simulink model "PicturePicture"  (R2015b)
settings: Solver=VariableStepAuto  StartTime=0.0  StopTime=500  RelTol=1e-3
libraries: simulink x4, powerlib_meascontrol x2
settings Model: Creator=ramin  LastModifiedBy=ramin

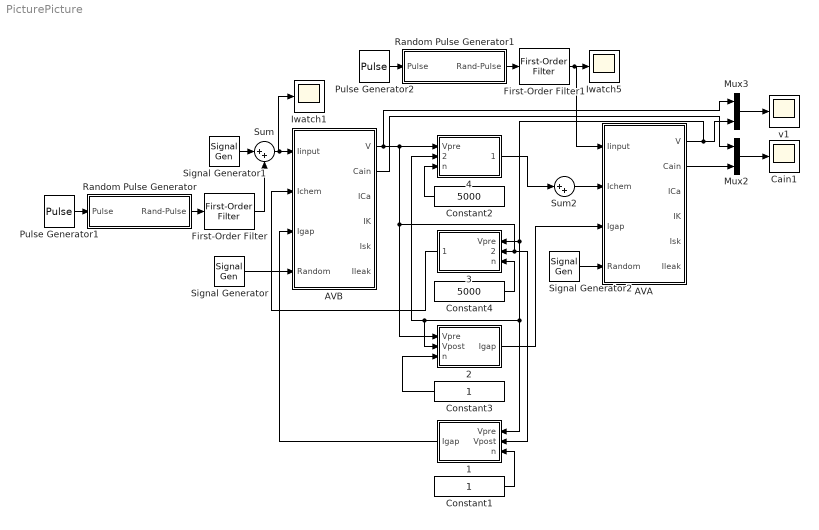
== system PicturePicture ==
  1 : Subsystem
  2 : Subsystem
  3 : Subsystem
  4 : Subsystem
  AVA : Subsystem
  AVB : Subsystem
  Cain1 : Scope
  Constant1 : Constant
  Constant2 : Constant  Value=5000
  Constant3 : Constant
  Constant4 : Constant  Value=5000
  First-Order Filter : powerlib_meascontrol/Filters/First-Order Filter  FilterType=Lowpass  Tc=1  Ts=0  Initialize=off  Vac_Init=[0, 0, 60]  Vdc_Init=0  PlotResponse=off  FreqRange="[0,  200,  1]"
  First-Order Filter1 : powerlib_meascontrol/Filters/First-Order Filter  FilterType=Lowpass  Tc=1  Ts=0  Initialize=off  Vac_Init=[0, 0, 60]  Vdc_Init=0  PlotResponse=off  FreqRange="[0,  200,  1]"
  Iwatch1 : Scope
  Iwatch5 : Scope
  Mux2 : Mux  Inputs=2
  Mux3 : Mux  Inputs=2
  Pulse Generator1 : DiscretePulseGenerator  PulseType=Time based  Amplitude=2000  Period=200  PulseWidth=80  PhaseDelay=2
  Pulse Generator2 : DiscretePulseGenerator  PulseType=Time based  Amplitude=2000  Period=200  PulseWidth=80  PhaseDelay=2
  Random Pulse Generator : Subsystem
  Random Pulse Generator1 : Subsystem
  Signal Generator : SignalGenerator  WaveForm=random  Amplitude=0.5  Frequency=100
  Signal Generator1 : SignalGenerator  WaveForm=random  Amplitude=0  Frequency=100
  Signal Generator2 : SignalGenerator  WaveForm=random  Amplitude=0.5  Frequency=100
  Sum : Sum  Inputs=|++
  Sum2 : Sum  Inputs=|++
  v1 : Scope
  wires:
  Signal Generator/1 -> AVB/4(Random)
  Signal Generator1/1 -> Sum/1
  Signal Generator2/1 -> AVA/4(Random)
  Constant2/1 -> 4/3(n)
  Constant3/1 -> 2/3(n)
  AVA/1(V) -> 1/1(Vpre), 2/2(Vpost), 4/2(Vpost), 3/1(Vpre), Mux3/2
  Sum/1 -> Iwatch1/1, AVB/1(Iinput)
  Random Pulse Generator/1(Rand-Pulse) -> First-Order Filter/1
  Sum2/1 -> AVA/2(Ichem)
  Constant1/1 -> 1/3(n)
  1/1(Igap) -> AVB/3(Igap)
  First-Order Filter1/1 -> AVA/1(Iinput), Iwatch5/1
  3/1(Ichem) -> AVB/2(Ichem)
  2/1(Igap) -> AVA/3(Igap)
  Mux2/1 -> Cain1/1
  Mux3/1 -> v1/1
  AVB/2("Cain ") -> Mux2/1
  4/1(Ichem) -> Sum2/1
  Pulse Generator1/1 -> Random Pulse Generator/1(Pulse)
  AVA/2("Cain ") -> Mux2/2
  Random Pulse Generator1/1(Rand-Pulse) -> First-Order Filter1/1
  Pulse Generator2/1 -> Random Pulse Generator1/1(Pulse)
  Constant4/1 -> 3/3(n)
  AVB/1(V) -> 4/1(Vpre), 2/1(Vpre), 1/2(Vpost), 3/2(Vpost), Mux3/1
  First-Order Filter/1 -> Sum/2

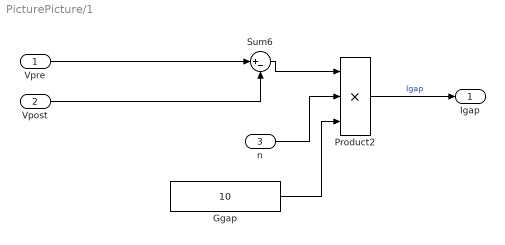
== system PicturePicture/1 ==
  Vpre : Inport
  Vpost : Inport  Port=2
  n : Inport  Port=3
  Ggap : Constant  Value=10
  Product2 : Product  Inputs=3
  Sum6 : Sum  Inputs=|+-
  Igap : Outport
  wires:
  Vpre/1 -> Sum6/1
  n/1 -> Product2/2
  Sum6/1 -> Product2/1
  Product2/1 -> Igap/1  "Igap"
  Vpost/1 -> Sum6/2
  Ggap/1 -> Product2/3

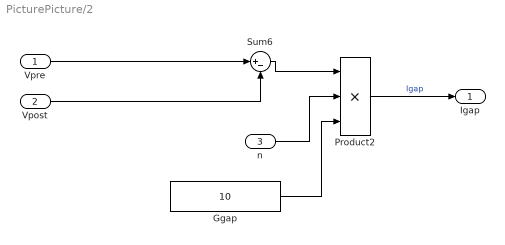
== system PicturePicture/2 ==
  Vpre : Inport
  Vpost : Inport  Port=2
  n : Inport  Port=3
  Ggap : Constant  Value=10
  Product2 : Product  Inputs=3
  Sum6 : Sum  Inputs=|+-
  Igap : Outport
  wires:
  Vpre/1 -> Sum6/1
  n/1 -> Product2/2
  Sum6/1 -> Product2/1
  Product2/1 -> Igap/1  "Igap"
  Vpost/1 -> Sum6/2
  Ggap/1 -> Product2/3

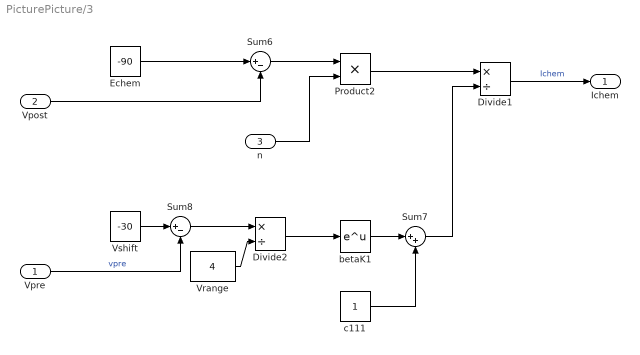
== system PicturePicture/3 ==
  Vpre : Inport
  Vpost : Inport  Port=2
  n : Inport  Port=3
  Divide1 : Product  Inputs=*/
  Divide2 : Product  Inputs=*/
  Echem : Constant  Value=-90
  Product2 : Product
  Sum6 : Sum  Inputs=|+-
  Sum7 : Sum  Inputs=|++
  Sum8 : Sum  Inputs=|+-
  Vrange : Constant  Value=4
  Vshift : Constant  Value=-30
  betaK1 : Math  SaturateOnIntegerOverflow=on
  c111 : Constant
  Ichem : Outport
  wires:
  Echem/1 -> Sum6/1
  n/1 -> Product2/2
  Sum6/1 -> Product2/1
  Product2/1 -> Divide1/1
  betaK1/1 -> Sum7/1
  c111/1 -> Sum7/2
  Vshift/1 -> Sum8/1
  Vpre/1 -> Sum8/2  "vpre"
  Sum8/1 -> Divide2/1
  Vrange/1 -> Divide2/2
  Divide2/1 -> betaK1/1
  Sum7/1 -> Divide1/2
  Divide1/1 -> Ichem/1  "Ichem"
  Vpost/1 -> Sum6/2

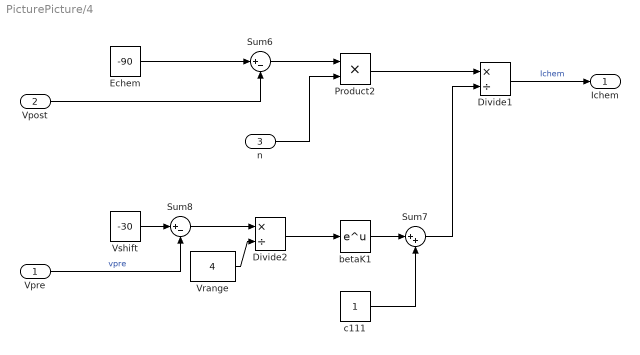
== system PicturePicture/4 ==
  Vpre : Inport
  Vpost : Inport  Port=2
  n : Inport  Port=3
  Divide1 : Product  Inputs=*/
  Divide2 : Product  Inputs=*/
  Echem : Constant  Value=-90
  Product2 : Product
  Sum6 : Sum  Inputs=|+-
  Sum7 : Sum  Inputs=|++
  Sum8 : Sum  Inputs=|+-
  Vrange : Constant  Value=4
  Vshift : Constant  Value=-30
  betaK1 : Math  SaturateOnIntegerOverflow=on
  c111 : Constant
  Ichem : Outport
  wires:
  Echem/1 -> Sum6/1
  n/1 -> Product2/2
  Sum6/1 -> Product2/1
  Product2/1 -> Divide1/1
  betaK1/1 -> Sum7/1
  c111/1 -> Sum7/2
  Vshift/1 -> Sum8/1
  Vpre/1 -> Sum8/2  "vpre"
  Sum8/1 -> Divide2/1
  Vrange/1 -> Divide2/2
  Divide2/1 -> betaK1/1
  Sum7/1 -> Divide1/2
  Divide1/1 -> Ichem/1  "Ichem"
  Vpost/1 -> Sum6/2

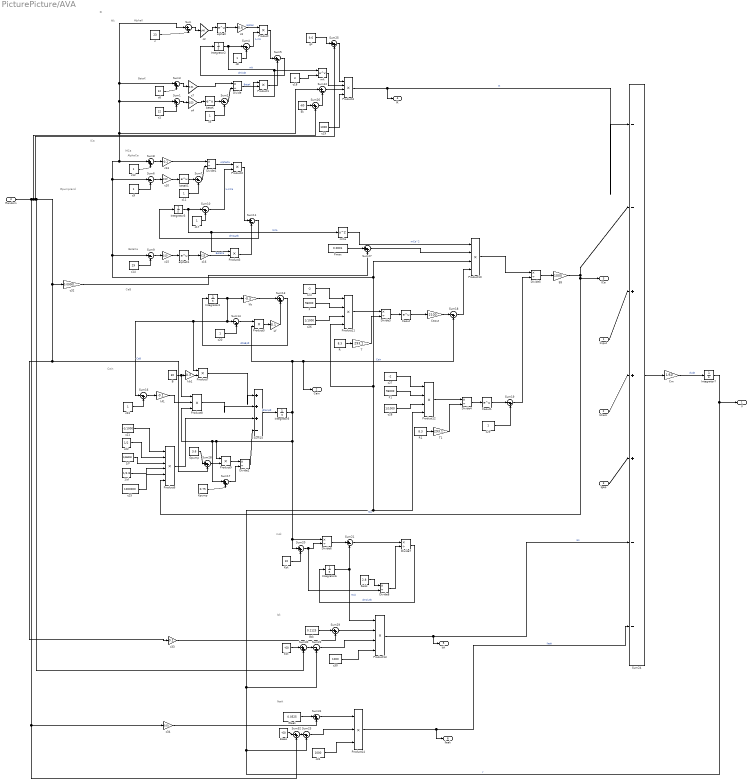
== system PicturePicture/AVA ==
  note: Gpumprand
  note: Isk
  note: msk
  note: ICa
  note: Cain
  note: CaB
  note: BetaCa
  note: AlphaCa
  note: MCa
  note: IK
  note: Mk
  note: BetaK
  note: AlphaK
  note: Ileak
  Iinput : Inport
  Ichem : Inport  Port=2
  Igap : Inport  Port=3
  Random : Inport  Port=4
  1/F : Constant  Value=1/96000
  1/d : Constant  Value=1/2.8
  B : Constant  Value=30
  Caout : Math  SaturateOnIntegerOverflow=on
  "Caout " : Gain  Gain=2100
  Caout1 : Math  SaturateOnIntegerOverflow=on
  "Cm " : Gain  Gain=1/50
  Divide{,1..8} (9 alike) : Product  Inputs=*/
  "Ek " : Constant  Value=-60
  Eleak : Constant  Value=-60
  Esk : Constant  Value=-60
  F : Constant  Value=96000
  F1 : Constant  Value=96000
  Gleak : Constant  Value=0.0525
  Gpump : Constant  Value=3.6
  Gsk : Constant  Value=0.2125
  Integrator2 : Integrator
  Integrator3 : Integrator  InitialCondition=0.001
  Integrator4 : Integrator
  Integrator5 : Integrator
  Integrator6 : Integrator  InitialCondition=1
  Integrator7 : Integrator  InitialCondition=-60
  Kpump : Constant  Value=0.75
  Ksk : Constant  Value=10
  Pmax : Constant  Value=0.0001
  Product{,1..3,5,7,9} (7 alike) : Product
  Product{4,10..13} (5 alike) : Product  Inputs=4
  Product14 : Product  Inputs=3
  Product6 : Product  Inputs=6
  Product8 : Product  Inputs=3
  R : Constant  Value=8.3
  R1 : Constant  Value=8.3
  Saisk : Constant  Value=2.8
  Sum{,2,5,7,11..12,21} (7 alike) : Sum  Inputs=|+-
  Sum{1,3,8,13,17,20,25..32} (14 alike) : Sum  Inputs=|++
  Sum{4,10,14,16,18..19,22..23} (8 alike) : Sum  Inputs=|-+
  Sum15 : Sum  Inputs=|+++-
  Sum24 : Sum  Inputs=|--+++--
  Sum6 : Sum  Inputs=|--
  Sum9 : Sum  Inputs=|--
  T : Gain  Gain=293.1
  T1 : Gain  Gain=293.1
  alphaK : Math  SaturateOnIntegerOverflow=on
  alphaK1 : Math  SaturateOnIntegerOverflow=on
  betaK : Math  SaturateOnIntegerOverflow=on
  betaK1 : Math  SaturateOnIntegerOverflow=on
  c : Constant  Value=23
  c1 : Constant  Value=12
  c10 : Gain  Gain=1/10
  c{5,8..9,11..12,17,20,23,29} (9 alike) : Constant
  c13 : Gain  Gain=-0.2
  c14 : Constant  Value=29
  c15 : Gain  Gain=1/10
  c16 : Gain  Gain=0.23
  c18 : Constant  Value=3
  c19 : Constant  Value=1000
  c2 : Gain  Gain=1/46
  c21 : Constant  Value=-1/1000
  c22 : Constant  Value=1/2
  c24 : Constant  Value=-2
  c25 : Constant  Value=1000000
  c26 : Constant  Value=1/1000
  c27 : Constant  Value=-2
  c28 : Constant  Value=1/1000
  c3 : Gain  Gain=0.6
  c30 : Constant  Value=1000
  c31 : Constant  Value=1000
  c32 : Gain  Gain=0.00001
  c33 : Gain  Gain=0.1
  c34 : Gain  Gain=0.01
  c4 : Gain  Gain=1/23
  c6 : Constant  Value=12
  c7 : Gain  Gain=0.01
  "gg " : Gain  Gain=1000
  gk : Constant  Value=9.6
  kb : Gain  Gain=-0.3
  kb1 : Gain  Gain=0.3
  kf : Gain  Gain=0.1
  kf1 : Gain  Gain=-0.1
  mCa : Math  Operator=square  SaturateOnIntegerOverflow=on
  mk : Math  Operator=pow  SaturateOnIntegerOverflow=on
  V : Outport
  "Cain " : Outport  Port=2
  ICa : Outport  Port=3
  IK : Outport  Port=4
  Isk : Outport  Port=5
  Ileak : Outport  Port=6
  wires:
  Divide/1 -> Product1/2  "BetaK"
  c10/1 -> betaK1/1
  Sum7/1 -> Divide1/2
  c/1 -> Sum/2
  R/1 -> T/1
  c3/1 -> Product/1  "alphaK"
  c9/1 -> Sum6/2
  c6/1 -> Sum3/2
  Product/1 -> Sum5/1
  Sum1/1 -> c4/1
  c13/1 -> Divide1/1
  Caout1/1 -> Sum19/1
  T/1 -> Divide3/2
  Ksk/1 -> Sum20/2
  Product14/1 -> Ileak/1, Sum24/7  "Ileak"
  Sum24/1 -> "Cm "/1
  "Cm "/1 -> Integrator7/1  "dv/dt"
  Divide3/1 -> Caout/1
  c31/1 -> Product14/3
  Integrator6/1 -> Sum21/2, Product13/1  "msk"
  Sum21/1 -> Divide7/1
  Sum23/1 -> Product14/2
  Divide6/1 -> Sum21/1
  c12/1 -> Sum8/2
  Integrator3/1 -> Product3/1, mCa/1, Sum10/1  "mCa"
  Sum5/1 -> Integrator2/1  "dmk/dt"
  c15/1 -> alphaK1/1
  Sum9/1 -> c15/1
  c2/1 -> alphaK/1
  Sum22/1 -> Product13/3
  Product10/1 -> Divide5/1
  Integrator2/1 -> mk/1, Product1/1, Sum4/1  "mk"
  Divide8/1 -> Divide7/2
  R1/1 -> T1/1
  Caout/1 -> "Caout "/1
  Sum3/1 -> c7/1
  Sum6/1 -> c10/1
  Divide4/1 -> Caout1/1
  c30/1 -> Product13/4
  c28/1 -> Product12/3
  c11/1 -> Sum7/2
  betaK1/1 -> Sum7/1
  Divide7/1 -> Integrator6/1  "dmsk/dt"
  Ichem/1 -> Sum24/4
  c7/1 -> Divide/1
  Sum14/1 -> Product5/1
  Sum13/1 -> Integrator4/1  "dCaB/dt"
  Integrator5/1 -> Sum20/1, Divide6/1, Product9/1, Sum17/1, Product8/3, "Cain "/1, Sum18/2, Product5/2  "Cain"
  c21/1 -> Product6/1
  c22/1 -> Product6/2
  1/F/1 -> Product6/3
  1/d/1 -> Product6/4
  c25/1 -> Product6/5
  "gg "/1 -> Sum24/2, ICa/1, Product6/6  "ICa"
  B/1 -> Product8/1, kb1/1
  kb1/1 -> Product7/2
  Product7/1 -> Sum15/1
  Product5/1 -> kf/1
  kf/1 -> Sum13/2
  c23/1 -> Sum16/2
  Sum16/1 -> kf1/1
  kf1/1 -> Product8/2
  Product8/1 -> Sum15/2
  Product6/1 -> Sum15/3
  Product9/1 -> Divide2/1
  Kpump/1 -> Sum17/2
  Sum17/1 -> Divide2/2
  Divide2/1 -> Sum15/4
  Sum15/1 -> Integrator5/1  "dCain/dt"
  mCa/1 -> Product10/1  "mCa^2"
  c24/1 -> Product11/1
  F/1 -> Product11/2
  c26/1 -> Product11/3
  Integrator7/1 -> V/1, Sum22/2, Product11/4, Product10/3, Sum6/1, Sum1/1, Sum3/1, Sum/1, Sum12/1, Sum8/1, Sum9/1, Product12/4, Sum23/2  "v"
  c14/1 -> Sum9/2
  Saisk/1 -> Divide8/1
  Sum18/1 -> Product10/4
  Iinput/1 -> Sum24/3
  "Caout "/1 -> Sum18/1
  Sum/1 -> c2/1
  Sum8/1 -> c13/1
  c16/1 -> Product3/2  "BetaCa"
  Product11/1 -> Divide3/1
  T1/1 -> Divide4/2
  betaK/1 -> Sum2/1
  c29/1 -> Sum19/2
  Product1/1 -> Sum5/2
  c4/1 -> betaK/1
  alphaK/1 -> c3/1
  alphaK1/1 -> c16/1
  Divide1/1 -> Product2/1  "AlphaCa"
  Sum2/1 -> Divide/2
  Sum4/1 -> Product/2  "1-mk"
  c5/1 -> Sum2/2
  c8/1 -> Sum4/2
  Igap/1 -> Sum24/5
  Product13/1 -> Isk/1, Sum24/6  "Isk"
  Divide5/1 -> "gg "/1
  Sum20/1 -> Divide8/2, Divide6/2
  Product12/1 -> Divide4/1
  c27/1 -> Product12/1
  F1/1 -> Product12/2
  c1/1 -> Sum1/2
  Sum11/1 -> Integrator3/1  "dmCa/dt"
  c17/1 -> Sum10/2
  "Ek "/1 -> Sum26/1
  Sum10/1 -> Product2/2  "1-mCa"
  Sum12/1 -> Product4/3
  Product3/1 -> Sum11/2
  Product4/1 -> IK/1, Sum24/1  "IK"
  Integrator4/1 -> Product7/1, Sum16/1, Sum14/1, kb/1  "CaB"
  kb/1 -> Sum13/1
  c20/1 -> Sum14/2
  mk/1 -> Product4/2
  Random/1 -> c32/1, c33/1, Sum28/2, Sum30/2, Sum25/2, Sum26/2, Sum32/2, c34/1
  c19/1 -> Product4/4
  Product2/1 -> Sum11/1
  c18/1 -> mk/2
  Sum19/1 -> Divide5/2
  gk/1 -> Sum25/1
  Sum25/1 -> Product4/1
  Sum26/1 -> Sum12/2
  Pmax/1 -> Sum27/1
  Sum27/1 -> Product10/2
  Sum28/1 -> Product9/2
  Gpump/1 -> Sum28/1
  Sum29/1 -> Product13/2
  Gsk/1 -> Sum29/1
  Sum30/1 -> Sum22/1
  Esk/1 -> Sum30/1
  Gleak/1 -> Sum31/1
  Sum31/1 -> Product14/1
  Sum32/1 -> Sum23/1
  Eleak/1 -> Sum32/1
  c32/1 -> Sum27/2
  c33/1 -> Sum29/2
  c34/1 -> Sum31/2

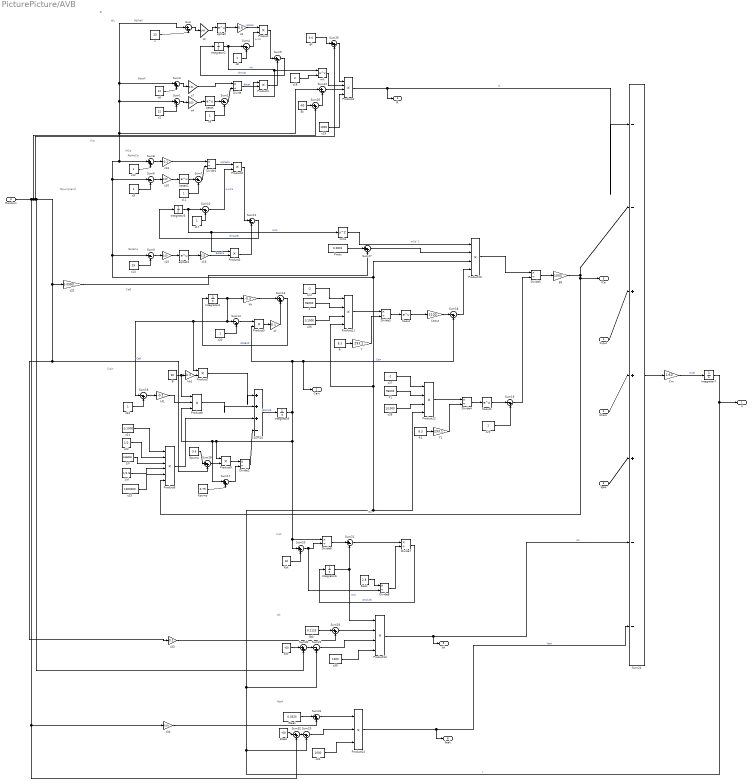
== system PicturePicture/AVB ==
  note: Gpumprand
  note: Isk
  note: msk
  note: ICa
  note: Cain
  note: CaB
  note: BetaCa
  note: AlphaCa
  note: MCa
  note: IK
  note: Mk
  note: BetaK
  note: AlphaK
  note: Ileak
  Iinput : Inport
  Ichem : Inport  Port=2
  Igap : Inport  Port=3
  Random : Inport  Port=4
  1/F : Constant  Value=1/96000
  1/d : Constant  Value=1/2.8
  B : Constant  Value=30
  Caout : Math  SaturateOnIntegerOverflow=on
  "Caout " : Gain  Gain=2100
  Caout1 : Math  SaturateOnIntegerOverflow=on
  "Cm " : Gain  Gain=1/50
  Divide{,1..8} (9 alike) : Product  Inputs=*/
  "Ek " : Constant  Value=-60
  Eleak : Constant  Value=-60
  Esk : Constant  Value=-60
  F : Constant  Value=96000
  F1 : Constant  Value=96000
  Gleak : Constant  Value=0.0525
  Gpump : Constant  Value=3.6
  Gsk : Constant  Value=0.2125
  Integrator2 : Integrator
  Integrator3 : Integrator  InitialCondition=0.001
  Integrator4 : Integrator
  Integrator5 : Integrator
  Integrator6 : Integrator  InitialCondition=1
  Integrator7 : Integrator  InitialCondition=-60
  Kpump : Constant  Value=0.75
  Ksk : Constant  Value=10
  Pmax : Constant  Value=0.0001
  Product{,1..3,5,7,9} (7 alike) : Product
  Product{4,10..13} (5 alike) : Product  Inputs=4
  Product14 : Product  Inputs=3
  Product6 : Product  Inputs=6
  Product8 : Product  Inputs=3
  R : Constant  Value=8.3
  R1 : Constant  Value=8.3
  Saisk : Constant  Value=2.8
  Sum{,2,5,7,11..12,21} (7 alike) : Sum  Inputs=|+-
  Sum{1,3,8,13,17,20,25..32} (14 alike) : Sum  Inputs=|++
  Sum{4,10,14,16,18..19,22..23} (8 alike) : Sum  Inputs=|-+
  Sum15 : Sum  Inputs=|+++-
  Sum24 : Sum  Inputs=|--+++--
  Sum6 : Sum  Inputs=|--
  Sum9 : Sum  Inputs=|--
  T : Gain  Gain=293.1
  T1 : Gain  Gain=293.1
  alphaK : Math  SaturateOnIntegerOverflow=on
  alphaK1 : Math  SaturateOnIntegerOverflow=on
  betaK : Math  SaturateOnIntegerOverflow=on
  betaK1 : Math  SaturateOnIntegerOverflow=on
  c : Constant  Value=23
  c1 : Constant  Value=12
  c10 : Gain  Gain=1/10
  c{5,8..9,11..12,17,20,23,29} (9 alike) : Constant
  c13 : Gain  Gain=-0.2
  c14 : Constant  Value=29
  c15 : Gain  Gain=1/10
  c16 : Gain  Gain=0.23
  c18 : Constant  Value=3
  c19 : Constant  Value=1000
  c2 : Gain  Gain=1/46
  c21 : Constant  Value=-1/1000
  c22 : Constant  Value=1/2
  c24 : Constant  Value=-2
  c25 : Constant  Value=1000000
  c26 : Constant  Value=1/1000
  c27 : Constant  Value=-2
  c28 : Constant  Value=1/1000
  c3 : Gain  Gain=0.6
  c30 : Constant  Value=1000
  c31 : Constant  Value=1000
  c32 : Gain  Gain=0.00001
  c33 : Gain  Gain=0.1
  c34 : Gain  Gain=0.01
  c4 : Gain  Gain=1/23
  c6 : Constant  Value=12
  c7 : Gain  Gain=0.01
  "gg " : Gain  Gain=1000
  gk : Constant  Value=9.6
  kb : Gain  Gain=-0.3
  kb1 : Gain  Gain=0.3
  kf : Gain  Gain=0.1
  kf1 : Gain  Gain=-0.1
  mCa : Math  Operator=square  SaturateOnIntegerOverflow=on
  mk : Math  Operator=pow  SaturateOnIntegerOverflow=on
  V : Outport
  "Cain " : Outport  Port=2
  ICa : Outport  Port=3
  IK : Outport  Port=4
  Isk : Outport  Port=5
  Ileak : Outport  Port=6
  wires:
  Divide/1 -> Product1/2  "BetaK"
  c10/1 -> betaK1/1
  Sum7/1 -> Divide1/2
  c/1 -> Sum/2
  R/1 -> T/1
  c3/1 -> Product/1  "alphaK"
  c9/1 -> Sum6/2
  c6/1 -> Sum3/2
  Product/1 -> Sum5/1
  Sum1/1 -> c4/1
  c13/1 -> Divide1/1
  Caout1/1 -> Sum19/1
  T/1 -> Divide3/2
  Ksk/1 -> Sum20/2
  Product14/1 -> Ileak/1, Sum24/7  "Ileak"
  Sum24/1 -> "Cm "/1
  "Cm "/1 -> Integrator7/1  "dv/dt"
  Divide3/1 -> Caout/1
  c31/1 -> Product14/3
  Integrator6/1 -> Sum21/2, Product13/1  "msk"
  Sum21/1 -> Divide7/1
  Sum23/1 -> Product14/2
  Divide6/1 -> Sum21/1
  c12/1 -> Sum8/2
  Integrator3/1 -> Product3/1, mCa/1, Sum10/1  "mCa"
  Sum5/1 -> Integrator2/1  "dmk/dt"
  c15/1 -> alphaK1/1
  Sum9/1 -> c15/1
  c2/1 -> alphaK/1
  Sum22/1 -> Product13/3
  Product10/1 -> Divide5/1
  Integrator2/1 -> mk/1, Product1/1, Sum4/1  "mk"
  Divide8/1 -> Divide7/2
  R1/1 -> T1/1
  Caout/1 -> "Caout "/1
  Sum3/1 -> c7/1
  Sum6/1 -> c10/1
  Divide4/1 -> Caout1/1
  c30/1 -> Product13/4
  c28/1 -> Product12/3
  c11/1 -> Sum7/2
  betaK1/1 -> Sum7/1
  Divide7/1 -> Integrator6/1  "dmsk/dt"
  Ichem/1 -> Sum24/4
  c7/1 -> Divide/1
  Sum14/1 -> Product5/1
  Sum13/1 -> Integrator4/1  "dCaB/dt"
  Integrator5/1 -> Sum20/1, Divide6/1, Product9/1, Sum17/1, Product8/3, "Cain "/1, Sum18/2, Product5/2  "Cain"
  c21/1 -> Product6/1
  c22/1 -> Product6/2
  1/F/1 -> Product6/3
  1/d/1 -> Product6/4
  c25/1 -> Product6/5
  "gg "/1 -> Sum24/2, ICa/1, Product6/6  "ICa"
  B/1 -> Product8/1, kb1/1
  kb1/1 -> Product7/2
  Product7/1 -> Sum15/1
  Product5/1 -> kf/1
  kf/1 -> Sum13/2
  c23/1 -> Sum16/2
  Sum16/1 -> kf1/1
  kf1/1 -> Product8/2
  Product8/1 -> Sum15/2
  Product6/1 -> Sum15/3
  Product9/1 -> Divide2/1
  Kpump/1 -> Sum17/2
  Sum17/1 -> Divide2/2
  Divide2/1 -> Sum15/4
  Sum15/1 -> Integrator5/1  "dCain/dt"
  mCa/1 -> Product10/1  "mCa^2"
  c24/1 -> Product11/1
  F/1 -> Product11/2
  c26/1 -> Product11/3
  Integrator7/1 -> V/1, Sum22/2, Product11/4, Product10/3, Sum6/1, Sum1/1, Sum3/1, Sum/1, Sum12/1, Sum8/1, Sum9/1, Product12/4, Sum23/2  "v"
  c14/1 -> Sum9/2
  Saisk/1 -> Divide8/1
  Sum18/1 -> Product10/4
  Iinput/1 -> Sum24/3
  "Caout "/1 -> Sum18/1
  Sum/1 -> c2/1
  Sum8/1 -> c13/1
  c16/1 -> Product3/2  "BetaCa"
  Product11/1 -> Divide3/1
  T1/1 -> Divide4/2
  betaK/1 -> Sum2/1
  c29/1 -> Sum19/2
  Product1/1 -> Sum5/2
  c4/1 -> betaK/1
  alphaK/1 -> c3/1
  alphaK1/1 -> c16/1
  Divide1/1 -> Product2/1  "AlphaCa"
  Sum2/1 -> Divide/2
  Sum4/1 -> Product/2  "1-mk"
  c5/1 -> Sum2/2
  c8/1 -> Sum4/2
  Igap/1 -> Sum24/5
  Product13/1 -> Isk/1, Sum24/6  "Isk"
  Divide5/1 -> "gg "/1
  Sum20/1 -> Divide8/2, Divide6/2
  Product12/1 -> Divide4/1
  c27/1 -> Product12/1
  F1/1 -> Product12/2
  c1/1 -> Sum1/2
  Sum11/1 -> Integrator3/1  "dmCa/dt"
  c17/1 -> Sum10/2
  "Ek "/1 -> Sum26/1
  Sum10/1 -> Product2/2  "1-mCa"
  Sum12/1 -> Product4/3
  Product3/1 -> Sum11/2
  Product4/1 -> IK/1, Sum24/1  "IK"
  Integrator4/1 -> Product7/1, Sum16/1, Sum14/1, kb/1  "CaB"
  kb/1 -> Sum13/1
  c20/1 -> Sum14/2
  mk/1 -> Product4/2
  Random/1 -> c32/1, c33/1, Sum28/2, Sum30/2, Sum25/2, Sum26/2, Sum32/2, c34/1
  c19/1 -> Product4/4
  Product2/1 -> Sum11/1
  c18/1 -> mk/2
  Sum19/1 -> Divide5/2
  gk/1 -> Sum25/1
  Sum25/1 -> Product4/1
  Sum26/1 -> Sum12/2
  Pmax/1 -> Sum27/1
  Sum27/1 -> Product10/2
  Sum28/1 -> Product9/2
  Gpump/1 -> Sum28/1
  Sum29/1 -> Product13/2
  Gsk/1 -> Sum29/1
  Sum30/1 -> Sum22/1
  Esk/1 -> Sum30/1
  Gleak/1 -> Sum31/1
  Sum31/1 -> Product14/1
  Sum32/1 -> Sum23/1
  Eleak/1 -> Sum32/1
  c32/1 -> Sum27/2
  c33/1 -> Sum29/2
  c34/1 -> Sum31/2

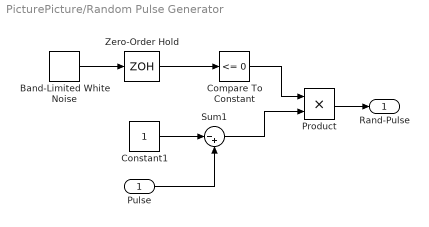
== system PicturePicture/Random Pulse Generator ==
  Pulse : Inport
  Band-Limited White Noise : simulink/Sources/Band-Limited White Noise  Cov=1  Ts=5  seed=15
  Compare To Constant : simulink/Logic and Bit Operations/Compare To Constant  relop=<=  const=0  OutDataTypeStr=boolean
  Constant1 : Constant
  Product : Product
  Sum1 : Sum  Inputs=|-+
  Zero-Order Hold : ZeroOrderHold  SampleTime=-1
  Rand-Pulse : Outport
  wires:
  Constant1/1 -> Sum1/1
  Sum1/1 -> Product/2
  Zero-Order Hold/1 -> Compare To Constant/1
  Product/1 -> Rand-Pulse/1
  Pulse/1 -> Sum1/2
  Band-Limited White Noise/1 -> Zero-Order Hold/1
  Compare To Constant/1 -> Product/1

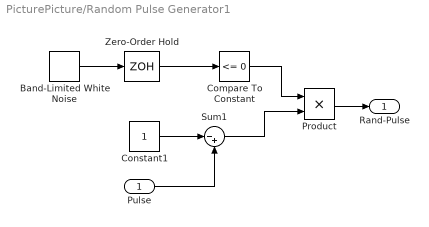
== system PicturePicture/Random Pulse Generator1 ==
  Pulse : Inport
  Band-Limited White Noise : simulink/Sources/Band-Limited White Noise  Cov=1  Ts=10  seed=20
  Compare To Constant : simulink/Logic and Bit Operations/Compare To Constant  relop=<=  const=0  OutDataTypeStr=boolean
  Constant1 : Constant
  Product : Product
  Sum1 : Sum  Inputs=|-+
  Zero-Order Hold : ZeroOrderHold  SampleTime=-1
  Rand-Pulse : Outport
  wires:
  Constant1/1 -> Sum1/1
  Sum1/1 -> Product/2
  Zero-Order Hold/1 -> Compare To Constant/1
  Product/1 -> Rand-Pulse/1
  Pulse/1 -> Sum1/2
  Band-Limited White Noise/1 -> Zero-Order Hold/1
  Compare To Constant/1 -> Product/1
